simulink model "motor_function"  (R2021a)
settings: configuration reference "motor_ctrl_config" (kept outside this file)
values from neighbouring files (symbols this model uses):
  sys_regs = 1    [motor_ctrl_data.sldd]
libraries: simulink x20
settings Model: DataDictionary=motor_ctrl_data.sldd  OrderedModelArguments=off  Creator=Litao  LastModifiedBy=Litao
settings ConfigSetRef: SourceName=motor_ctrl_config

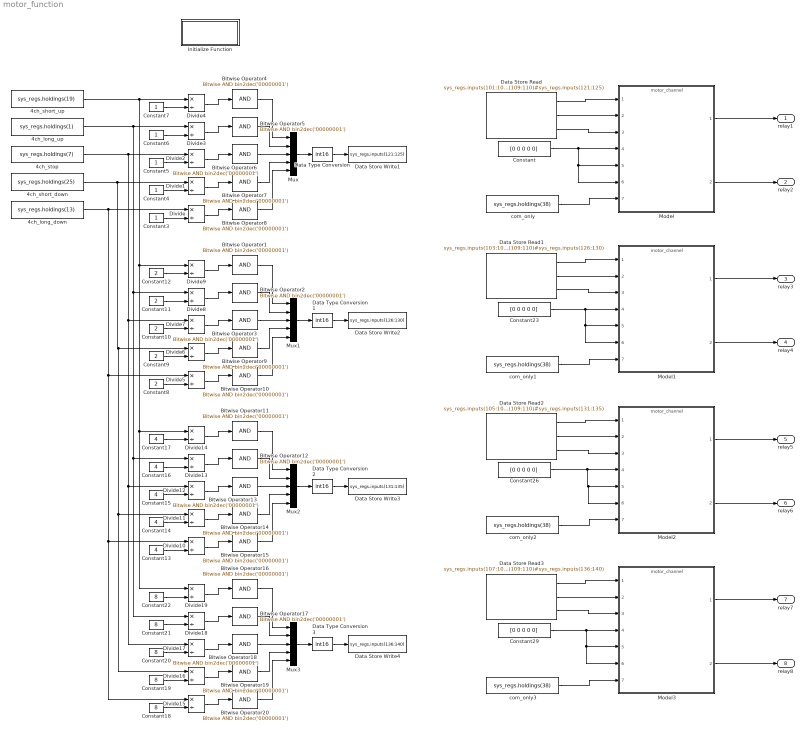
== system motor_function ==
  4ch_long_down : DataStoreRead  DataStoreName=sys_regs  DataStoreElements=sys_regs.holdings(13)  IndexOptions=Index vector (dialog)  Indices=1  OutputSizes=1
  4ch_long_up : DataStoreRead  DataStoreName=sys_regs  DataStoreElements=sys_regs.holdings(1)  IndexOptions=Index vector (dialog)  Indices=1  OutputSizes=1
  4ch_short_down : DataStoreRead  DataStoreName=sys_regs  DataStoreElements=sys_regs.holdings(25)  IndexOptions=Index vector (dialog)  Indices=1  OutputSizes=1
  4ch_short_up : DataStoreRead  DataStoreName=sys_regs  DataStoreElements=sys_regs.holdings(19)  IndexOptions=Index vector (dialog)  Indices=1  OutputSizes=1
  4ch_stop : DataStoreRead  DataStoreName=sys_regs  DataStoreElements=sys_regs.holdings(7)  IndexOptions=Index vector (dialog)  Indices=1  OutputSizes=1
  Bitwise Operator{1..20} (20 alike) : simulink/Logic and Bit Operations/Bitwise Operator  logicop=AND  UseBitMask=on  BitMask=bin2dec('00000001')  BitMaskRealWorld=Stored Integer
  Constant{,23,26,29} (4 alike) : Constant  Value=[0 0 0 0 0]  OutDataTypeStr=int16
  Constant{8..12} (5 alike) : Constant  Value=2  OutDataTypeStr=int16
  Constant{13..17} (5 alike) : Constant  Value=4  OutDataTypeStr=int16
  Constant{18..22} (5 alike) : Constant  Value=8  OutDataTypeStr=int16
  Constant{3..7} (5 alike) : Constant  OutDataTypeStr=int16
  Data Store Read : DataStoreRead  DataStoreName=sys_regs  DataStoreElements=sys_regs.inputs(101:102)#sys_regs.inputs(109:110)#sys_regs.inputs(121:125)  IndexOptions=Index vector (dialog)  Indices=1  OutputSizes=1
  Data Store Read1 : DataStoreRead  DataStoreName=sys_regs  DataStoreElements=sys_regs.inputs(103:104)#sys_regs.inputs(109:110)#sys_regs.inputs(126:130)  IndexOptions=Index vector (dialog)  Indices=1  OutputSizes=1
  Data Store Read2 : DataStoreRead  DataStoreName=sys_regs  DataStoreElements=sys_regs.inputs(105:106)#sys_regs.inputs(109:110)#sys_regs.inputs(131:135)  IndexOptions=Index vector (dialog)  Indices=1  OutputSizes=1
  Data Store Read3 : DataStoreRead  DataStoreName=sys_regs  DataStoreElements=sys_regs.inputs(107:108)#sys_regs.inputs(109:110)#sys_regs.inputs(136:140)  IndexOptions=Index vector (dialog)  Indices=1  OutputSizes=1
  Data Store Write1 : DataStoreWrite  DataStoreName=sys_regs  DataStoreElements=sys_regs.inputs(121:125)  IndexOptions=Index vector (dialog)  Indices=1  OutputSizes=1
  Data Store Write2 : DataStoreWrite  DataStoreName=sys_regs  DataStoreElements=sys_regs.inputs(126:130)  IndexOptions=Index vector (dialog)  Indices=1  OutputSizes=1
  Data Store Write3 : DataStoreWrite  DataStoreName=sys_regs  DataStoreElements=sys_regs.inputs(131:135)  IndexOptions=Index vector (dialog)  Indices=1  OutputSizes=1
  Data Store Write4 : DataStoreWrite  DataStoreName=sys_regs  DataStoreElements=sys_regs.inputs(136:140)  IndexOptions=Index vector (dialog)  Indices=1  OutputSizes=1
  Data Type Conversion{,1..3} (4 alike) : DataTypeConversion  OutDataTypeStr=int16
  Divide{,1..19} (20 alike) : Product  Inputs=*/  OutDataTypeStr=int16
  Initialize Function : Subsystem  TreatAsAtomicUnit=on
  Model{,1..3} (4 alike) : ModelReference  ModelNameDialog=motor_channel.slx  UsingDefaultArgumentValue=0,0,0,0,0  SimulationMode=Normal  ModelReferenceVersion=1.11
  Mux{,1..3} (4 alike) : Mux  Inputs=5
  com_only{,1..3} (4 alike) : DataStoreRead  DataStoreName=sys_regs  DataStoreElements=sys_regs.holdings(38)  IndexOptions=Index vector (dialog)  Indices=1  OutputSizes=1
  relay1 : Outport
  relay2 : Outport  Port=2
  relay3 : Outport  Port=3
  relay4 : Outport  Port=4
  relay5 : Outport  Port=5
  relay6 : Outport  Port=6
  relay7 : Outport  Port=7
  relay8 : Outport  Port=8
  wires:
  Data Store Read/1 -> Model/1
  Model/1 -> relay1/1
  Model/2 -> relay2/1
  Bitwise Operator4/1 -> Mux/1
  Bitwise Operator5/1 -> Mux/2
  Bitwise Operator6/1 -> Mux/3
  Bitwise Operator7/1 -> Mux/4
  Bitwise Operator8/1 -> Mux/5
  Mux/1 -> Data Type Conversion/1
  Constant/1 -> Model/6, Model/5, Model/4
  Data Store Read/2 -> Model/2
  Constant3/1 -> Divide/2
  4ch_long_down/1 -> Divide15/1, Divide10/1, Divide5/1, Divide/1
  Divide/1 -> Bitwise Operator8/1
  Constant4/1 -> Divide1/2
  Constant5/1 -> Divide2/2
  Constant6/1 -> Divide3/2
  Constant7/1 -> Divide4/2
  4ch_short_up/1 -> Divide19/1, Divide14/1, Divide9/1, Divide4/1
  Divide4/1 -> Bitwise Operator4/1
  4ch_long_up/1 -> Divide18/1, Divide13/1, Divide8/1, Divide3/1
  Divide3/1 -> Bitwise Operator5/1
  4ch_stop/1 -> Divide17/1, Divide12/1, Divide7/1, Divide2/1
  Divide2/1 -> Bitwise Operator6/1
  Divide1/1 -> Bitwise Operator7/1
  4ch_short_down/1 -> Divide16/1, Divide11/1, Divide6/1, Divide1/1
  Data Type Conversion/1 -> Data Store Write1/1
  com_only/1 -> Model/7
  Data Store Read/3 -> Model/3
  Divide6/1 -> Bitwise Operator9/1
  Constant11/1 -> Divide8/2
  Divide7/1 -> Bitwise Operator3/1
  Constant10/1 -> Divide7/2
  Constant9/1 -> Divide6/2
  Divide9/1 -> Bitwise Operator1/1
  Constant12/1 -> Divide9/2
  Divide5/1 -> Bitwise Operator10/1
  Divide8/1 -> Bitwise Operator2/1
  Constant8/1 -> Divide5/2
  Divide11/1 -> Bitwise Operator14/1
  Constant16/1 -> Divide13/2
  Divide12/1 -> Bitwise Operator13/1
  Constant15/1 -> Divide12/2
  Constant14/1 -> Divide11/2
  Divide14/1 -> Bitwise Operator11/1
  Constant17/1 -> Divide14/2
  Divide10/1 -> Bitwise Operator15/1
  Divide13/1 -> Bitwise Operator12/1
  Constant13/1 -> Divide10/2
  Divide16/1 -> Bitwise Operator19/1
  Constant21/1 -> Divide18/2
  Divide17/1 -> Bitwise Operator18/1
  Constant20/1 -> Divide17/2
  Constant19/1 -> Divide16/2
  Divide19/1 -> Bitwise Operator16/1
  Constant22/1 -> Divide19/2
  Divide15/1 -> Bitwise Operator20/1
  Divide18/1 -> Bitwise Operator17/1
  Constant18/1 -> Divide15/2
  Data Type Conversion1/1 -> Data Store Write2/1
  Mux1/1 -> Data Type Conversion1/1
  Bitwise Operator10/1 -> Mux1/5
  Bitwise Operator9/1 -> Mux1/4
  Bitwise Operator3/1 -> Mux1/3
  Bitwise Operator2/1 -> Mux1/2
  Bitwise Operator1/1 -> Mux1/1
  Bitwise Operator11/1 -> Mux2/1
  Bitwise Operator12/1 -> Mux2/2
  Bitwise Operator13/1 -> Mux2/3
  Bitwise Operator14/1 -> Mux2/4
  Bitwise Operator15/1 -> Mux2/5
  Mux2/1 -> Data Type Conversion2/1
  Data Type Conversion2/1 -> Data Store Write3/1
  Data Type Conversion3/1 -> Data Store Write4/1
  Mux3/1 -> Data Type Conversion3/1
  Bitwise Operator20/1 -> Mux3/5
  Bitwise Operator19/1 -> Mux3/4
  Bitwise Operator18/1 -> Mux3/3
  Bitwise Operator17/1 -> Mux3/2
  Bitwise Operator16/1 -> Mux3/1
  com_only1/1 -> Model1/7
  Constant23/1 -> Model1/6, Model1/5, Model1/4
  Model1/2 -> relay4/1
  Model1/1 -> relay3/1
  Data Store Read1/1 -> Model1/1
  Data Store Read1/2 -> Model1/2
  Data Store Read1/3 -> Model1/3
  com_only2/1 -> Model2/7
  Constant26/1 -> Model2/6, Model2/5, Model2/4
  Model2/2 -> relay6/1
  Model2/1 -> relay5/1
  Data Store Read2/1 -> Model2/1
  Data Store Read2/2 -> Model2/2
  Data Store Read2/3 -> Model2/3
  com_only3/1 -> Model3/7
  Constant29/1 -> Model3/6, Model3/5, Model3/4
  Model3/2 -> relay8/1
  Model3/1 -> relay7/1
  Data Store Read3/1 -> Model3/1
  Data Store Read3/2 -> Model3/2
  Data Store Read3/3 -> Model3/3

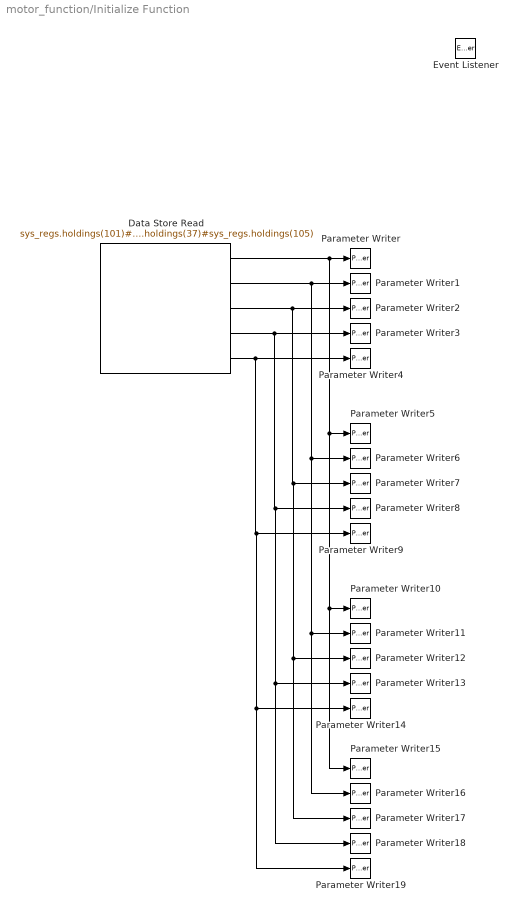
== system motor_function/Initialize Function ==
  Data Store Read : DataStoreRead  DataStoreName=sys_regs  DataStoreElements=sys_regs.holdings(101)#sys_regs.holdings(102)#sys_regs.holdings(103)#sys_regs.holdings(37)#sys_regs.holdings(105)  IndexOptions=Index vector (dialog)  Indices=1  OutputSizes=1
  Event Listener : EventListener  DisableCoverage=on  EventName=reset
  Parameter Writer : ParameterWriter  ParameterOwnerBlock=../../Model  ParameterName=debounce_cnt  ParameterInternalName=debounce_cnt
  Parameter Writer1 : ParameterWriter  ParameterOwnerBlock=../../Model  ParameterName=longpress_cnt  ParameterInternalName=longpress_cnt
  Parameter Writer10 : ParameterWriter  ParameterOwnerBlock=../../Model2  ParameterName=debounce_cnt  ParameterInternalName=debounce_cnt
  Parameter Writer11 : ParameterWriter  ParameterOwnerBlock=../../Model2  ParameterName=longpress_cnt  ParameterInternalName=longpress_cnt
  Parameter Writer12 : ParameterWriter  ParameterOwnerBlock=../../Model2  ParameterName=long_cnt  ParameterInternalName=long_cnt
  Parameter Writer13 : ParameterWriter  ParameterOwnerBlock=../../Model2  ParameterName=short_cnt  ParameterInternalName=short_cnt
  Parameter Writer14 : ParameterWriter  ParameterOwnerBlock=../../Model2  ParameterName=transfer_cnt  ParameterInternalName=transfer_cnt
  Parameter Writer15 : ParameterWriter  ParameterOwnerBlock=../../Model3  ParameterName=debounce_cnt  ParameterInternalName=debounce_cnt
  Parameter Writer16 : ParameterWriter  ParameterOwnerBlock=../../Model3  ParameterName=longpress_cnt  ParameterInternalName=longpress_cnt
  Parameter Writer17 : ParameterWriter  ParameterOwnerBlock=../../Model3  ParameterName=long_cnt  ParameterInternalName=long_cnt
  Parameter Writer18 : ParameterWriter  ParameterOwnerBlock=../../Model3  ParameterName=short_cnt  ParameterInternalName=short_cnt
  Parameter Writer19 : ParameterWriter  ParameterOwnerBlock=../../Model3  ParameterName=transfer_cnt  ParameterInternalName=transfer_cnt
  Parameter Writer2 : ParameterWriter  ParameterOwnerBlock=../../Model  ParameterName=long_cnt  ParameterInternalName=long_cnt
  Parameter Writer3 : ParameterWriter  ParameterOwnerBlock=../../Model  ParameterName=short_cnt  ParameterInternalName=short_cnt
  Parameter Writer4 : ParameterWriter  ParameterOwnerBlock=../../Model  ParameterName=transfer_cnt  ParameterInternalName=transfer_cnt
  Parameter Writer5 : ParameterWriter  ParameterOwnerBlock=../../Model1  ParameterName=debounce_cnt  ParameterInternalName=debounce_cnt
  Parameter Writer6 : ParameterWriter  ParameterOwnerBlock=../../Model1  ParameterName=longpress_cnt  ParameterInternalName=longpress_cnt
  Parameter Writer7 : ParameterWriter  ParameterOwnerBlock=../../Model1  ParameterName=long_cnt  ParameterInternalName=long_cnt
  Parameter Writer8 : ParameterWriter  ParameterOwnerBlock=../../Model1  ParameterName=short_cnt  ParameterInternalName=short_cnt
  Parameter Writer9 : ParameterWriter  ParameterOwnerBlock=../../Model1  ParameterName=transfer_cnt  ParameterInternalName=transfer_cnt
  wires:
  Data Store Read/1 -> Parameter Writer15/1, Parameter Writer10/1, Parameter Writer5/1, Parameter Writer/1
  Data Store Read/2 -> Parameter Writer16/1, Parameter Writer11/1, Parameter Writer6/1, Parameter Writer1/1
  Data Store Read/3 -> Parameter Writer17/1, Parameter Writer12/1, Parameter Writer7/1, Parameter Writer2/1
  Data Store Read/4 -> Parameter Writer18/1, Parameter Writer13/1, Parameter Writer8/1, Parameter Writer3/1
  Data Store Read/5 -> Parameter Writer19/1, Parameter Writer14/1, Parameter Writer9/1, Parameter Writer4/1
